simulink model "BlockTypeFrequencyAnalyzerTest"  (Simulink 6.3)
settings: Solver=ode45  StartTime=0.0  StopTime=10.0  RelTol=1e-3
undefined symbols (not defined in the file): DiscIntNeverNeededParam, NumBits1, NumBits2, sigbuilder_block, Slope1, Slope2
libraries: simulink x99
settings Model: LastModifiedBy=deissenb  BufferReuse=off
settings OptimizationCC: BlockReduction=off  InlineParams=on  BufferReuse=off

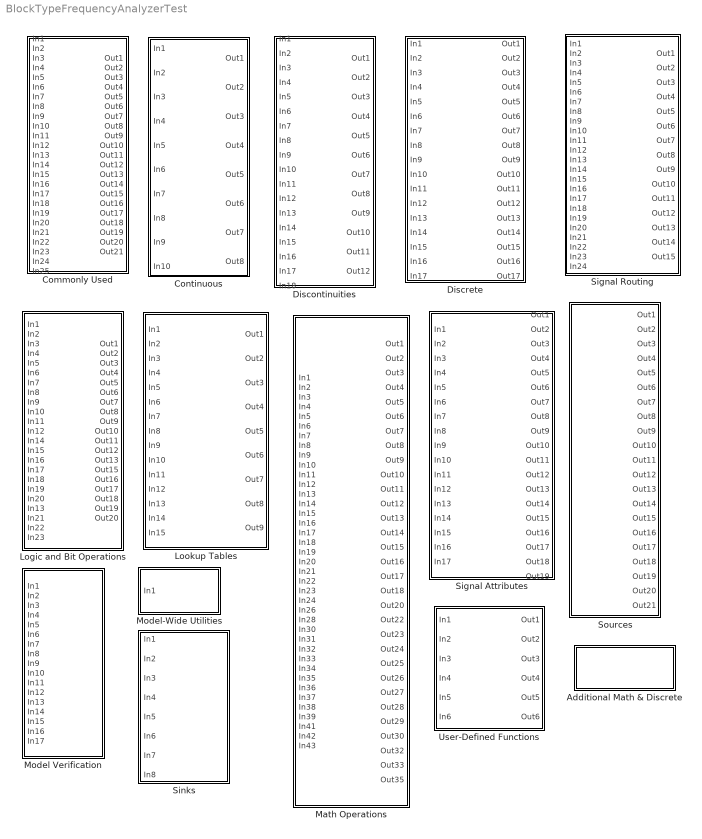
== system BlockTypeFrequencyAnalyzerTest ==
  Additional Math & Discrete : Subsystem
  Commonly Used : Subsystem
  Continuous : Subsystem
  Discontinuities : Subsystem
  Discrete : Subsystem
  Logic and Bit Operations : Subsystem
  Lookup Tables : Subsystem
  Math Operations : Subsystem
  Model Verification : Subsystem
  Model-Wide Utilities : Subsystem
  Signal Attributes : Subsystem
  Signal Routing : Subsystem
  Sinks : Subsystem
  Sources : Subsystem
  User-Defined Functions : Subsystem

== system BlockTypeFrequencyAnalyzerTest/Additional Math & Discrete ==
  Additional Discrete : Subsystem
  Additional Math : Subsystem

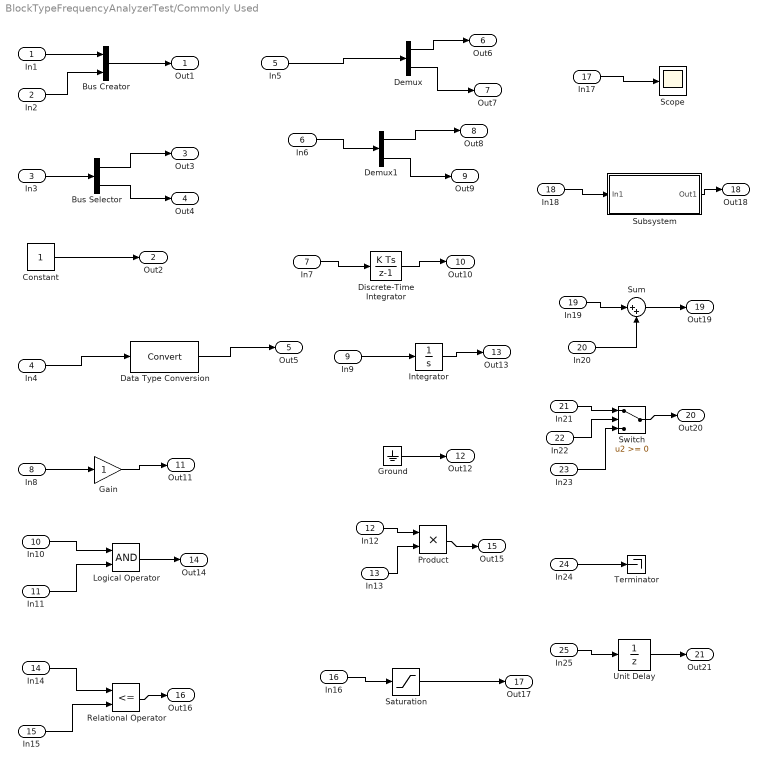
== system BlockTypeFrequencyAnalyzerTest/Commonly Used ==
  In1 : Inport
  In2 : Inport  Port=2
  In3 : Inport  Port=3
  In4 : Inport  Port=4
  In5 : Inport  Port=5
  In6 : Inport  Port=6
  In7 : Inport  Port=7
  In8 : Inport  Port=8
  In9 : Inport  Port=9
  In10 : Inport  Port=10
  In11 : Inport  Port=11
  In12 : Inport  Port=12
  In13 : Inport  Port=13
  In14 : Inport  Port=14
  In15 : Inport  Port=15
  In16 : Inport  Port=16
  In17 : Inport  Port=17
  In18 : Inport  Port=18
  In19 : Inport  Port=19
  In20 : Inport  Port=20
  In21 : Inport  Port=21
  In22 : Inport  Port=22
  In23 : Inport  Port=23
  In24 : Inport  Port=24
  In25 : Inport  Port=25
  Bus Creator : BusCreator  Inputs=2
  Bus Selector : BusSelector  OutputSignals=signal1,signal2
  Constant : Constant
  Data Type Conversion : DataTypeConversion
  Demux : Demux  Outputs=2
  Demux1 : Demux  Outputs=2
  Discrete-Time Integrator : DiscreteIntegrator  ICPrevOutput=DiscIntNeverNeededParam  ICPrevScaledInput=DiscIntNeverNeededParam
  Gain : Gain
  Ground : Ground
  Integrator : Integrator
  Logical Operator : Logic  AllPortsSameDT=off  OutDataTypeMode=Boolean
  Product : Product  RndMeth=Zero
  Relational Operator : RelationalOperator  Operator=<=  LogicOutDataTypeMode=Boolean
  Saturation : Saturate
  Scope : Scope
  Subsystem : Subsystem
  Sum : Sum  Inputs=|++
  Switch : Switch
  Terminator : Terminator
  Unit Delay : UnitDelay
  Out1 : Outport
  Out2 : Outport  Port=2
  Out3 : Outport  Port=3
  Out4 : Outport  Port=4
  Out5 : Outport  Port=5
  Out6 : Outport  Port=6
  Out7 : Outport  Port=7
  Out8 : Outport  Port=8
  Out9 : Outport  Port=9
  Out10 : Outport  Port=10
  Out11 : Outport  Port=11
  Out12 : Outport  Port=12
  Out13 : Outport  Port=13
  Out14 : Outport  Port=14
  Out15 : Outport  Port=15
  Out16 : Outport  Port=16
  Out17 : Outport  Port=17
  Out18 : Outport  Port=18
  Out19 : Outport  Port=19
  Out20 : Outport  Port=20
  Out21 : Outport  Port=21
  wires:
  Unit Delay/1 -> Out21/1
  In25/1 -> Unit Delay/1
  In24/1 -> Terminator/1
  Switch/1 -> Out20/1
  In23/1 -> Switch/3
  In22/1 -> Switch/2
  In21/1 -> Switch/1
  Sum/1 -> Out19/1
  In20/1 -> Sum/2
  In19/1 -> Sum/1
  Subsystem/1(Out1) -> Out18/1
  In18/1 -> Subsystem/1(In1)
  In17/1 -> Scope/1
  Saturation/1 -> Out17/1
  In16/1 -> Saturation/1
  Relational Operator/1 -> Out16/1
  In15/1 -> Relational Operator/2
  In14/1 -> Relational Operator/1
  Product/1 -> Out15/1
  In13/1 -> Product/2
  In12/1 -> Product/1
  Logical Operator/1 -> Out14/1
  In11/1 -> Logical Operator/2
  In10/1 -> Logical Operator/1
  Integrator/1 -> Out13/1
  In9/1 -> Integrator/1
  Ground/1 -> Out12/1
  Gain/1 -> Out11/1
  In8/1 -> Gain/1
  Discrete-Time Integrator/1 -> Out10/1
  In7/1 -> Discrete-Time Integrator/1
  Demux1/2 -> Out9/1
  Demux1/1 -> Out8/1
  In6/1 -> Demux1/1
  Demux/2 -> Out7/1
  Demux/1 -> Out6/1
  In5/1 -> Demux/1
  Data Type Conversion/1 -> Out5/1
  In4/1 -> Data Type Conversion/1
  Bus Selector/2 -> Out4/1
  Bus Selector/1 -> Out3/1
  In3/1 -> Bus Selector/1
  Constant/1 -> Out2/1
  Bus Creator/1 -> Out1/1
  In2/1 -> Bus Creator/2
  In1/1 -> Bus Creator/1

== system BlockTypeFrequencyAnalyzerTest/Continuous ==
  In1 : Inport
  In2 : Inport  Port=2
  In3 : Inport  Port=3
  In4 : Inport  Port=4
  In5 : Inport  Port=5
  In6 : Inport  Port=6
  In7 : Inport  Port=7
  In8 : Inport  Port=8
  In9 : Inport  Port=9
  In10 : Inport  Port=10
  Derivative : Derivative
  Integrator : Integrator
  State-Space : StateSpace
  Transfer Fcn : TransferFcn  Denominator=[1 1]
  Transport Delay : TransportDelay
  Variable Time Delay : VariableTransportDelay  MaximumDelay=10
  Variable Transport Delay : VariableTransportDelay  VariableDelayType=Variable transport delay  MaximumDelay=10
  Zero-Pole : ZeroPole  Poles=[0 -1]
  Out1 : Outport
  Out2 : Outport  Port=2
  Out3 : Outport  Port=3
  Out4 : Outport  Port=4
  Out5 : Outport  Port=5
  Out6 : Outport  Port=6
  Out7 : Outport  Port=7
  Out8 : Outport  Port=8
  wires:
  In1/1 -> Derivative/1
  In2/1 -> Integrator/1
  In3/1 -> State-Space/1
  In4/1 -> Transfer Fcn/1
  In5/1 -> Transport Delay/1
  In6/1 -> Variable Time Delay/1
  In7/1 -> Variable Time Delay/2
  In8/1 -> Variable Transport Delay/1
  In9/1 -> Variable Transport Delay/2
  In10/1 -> Zero-Pole/1
  Derivative/1 -> Out1/1
  Integrator/1 -> Out2/1
  State-Space/1 -> Out3/1
  Transfer Fcn/1 -> Out4/1
  Transport Delay/1 -> Out5/1
  Variable Time Delay/1 -> Out6/1
  Variable Transport Delay/1 -> Out7/1
  Zero-Pole/1 -> Out8/1

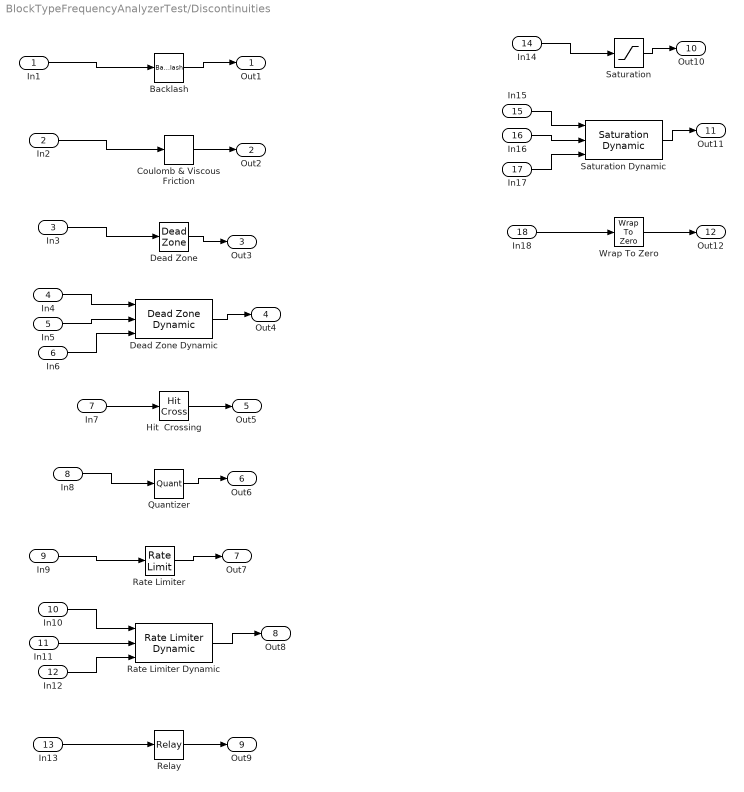
== system BlockTypeFrequencyAnalyzerTest/Discontinuities ==
  In1 : Inport
  In2 : Inport  Port=2
  In3 : Inport  Port=3
  In4 : Inport  Port=4
  In5 : Inport  Port=5
  In6 : Inport  Port=6
  In7 : Inport  Port=7
  In8 : Inport  Port=8
  In9 : Inport  Port=9
  In10 : Inport  Port=10
  In11 : Inport  Port=11
  In12 : Inport  Port=12
  In13 : Inport  Port=13
  In14 : Inport  Port=14
  In15 : Inport  Port=15
  In16 : Inport  Port=16
  In17 : Inport  Port=17
  In18 : Inport  Port=18
  Backlash : Backlash
  Coulomb & Viscous Friction : simulink/Discontinuities/Coulomb & Viscous Friction  offset=[1 3 2 0]  gain=1
  Dead Zone : DeadZone  SaturateOnIntegerOverflow=on
  Dead Zone Dynamic : simulink/Discontinuities/Dead Zone Dynamic
  Hit  Crossing : HitCross
  Quantizer : Quantizer
  Rate Limiter : RateLimiter  SampleTimeMode=inherited
  Rate Limiter Dynamic : simulink/Discontinuities/Rate Limiter Dynamic
  Relay : Relay
  Saturation : Saturate
  Saturation Dynamic : simulink/Discontinuities/Saturation Dynamic
  Wrap To Zero : simulink/Discontinuities/Wrap To Zero  Threshold=255
  Out1 : Outport
  Out2 : Outport  Port=2
  Out3 : Outport  Port=3
  Out4 : Outport  Port=4
  Out5 : Outport  Port=5
  Out6 : Outport  Port=6
  Out7 : Outport  Port=7
  Out8 : Outport  Port=8
  Out9 : Outport  Port=9
  Out10 : Outport  Port=10
  Out11 : Outport  Port=11
  Out12 : Outport  Port=12
  wires:
  In1/1 -> Backlash/1
  In2/1 -> Coulomb & Viscous Friction/1
  In3/1 -> Dead Zone/1
  In4/1 -> Dead Zone Dynamic/1
  In5/1 -> Dead Zone Dynamic/2
  In6/1 -> Dead Zone Dynamic/3
  In7/1 -> Hit  Crossing/1
  In8/1 -> Quantizer/1
  In9/1 -> Rate Limiter/1
  In10/1 -> Rate Limiter Dynamic/1
  In11/1 -> Rate Limiter Dynamic/2
  In12/1 -> Rate Limiter Dynamic/3
  In13/1 -> Relay/1
  In14/1 -> Saturation/1
  In15/1 -> Saturation Dynamic/1
  In16/1 -> Saturation Dynamic/2
  In17/1 -> Saturation Dynamic/3
  In18/1 -> Wrap To Zero/1
  Backlash/1 -> Out1/1
  Coulomb & Viscous Friction/1 -> Out2/1
  Dead Zone/1 -> Out3/1
  Dead Zone Dynamic/1 -> Out4/1
  Hit  Crossing/1 -> Out5/1
  Quantizer/1 -> Out6/1
  Rate Limiter/1 -> Out7/1
  Rate Limiter Dynamic/1 -> Out8/1
  Relay/1 -> Out9/1
  Saturation/1 -> Out10/1
  Saturation Dynamic/1 -> Out11/1
  Wrap To Zero/1 -> Out12/1

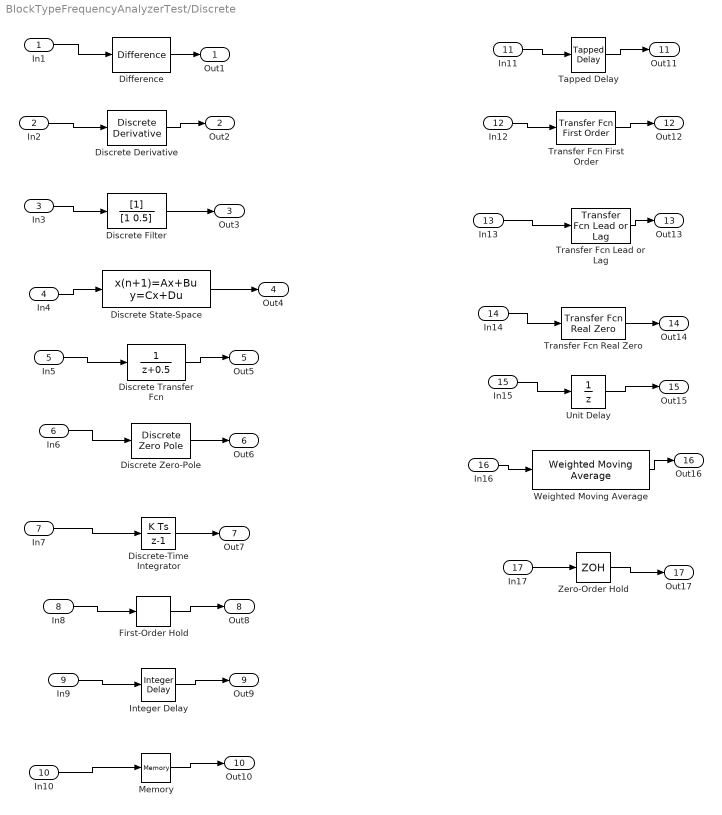
== system BlockTypeFrequencyAnalyzerTest/Discrete ==
  In1 : Inport
  In2 : Inport  Port=2
  In3 : Inport  Port=3
  In4 : Inport  Port=4
  In5 : Inport  Port=5
  In6 : Inport  Port=6
  In7 : Inport  Port=7
  In8 : Inport  Port=8
  In9 : Inport  Port=9
  In10 : Inport  Port=10
  In11 : Inport  Port=11
  In12 : Inport  Port=12
  In13 : Inport  Port=13
  In14 : Inport  Port=14
  In15 : Inport  Port=15
  In16 : Inport  Port=16
  In17 : Inport  Port=17
  Difference : simulink/Discrete/Difference  ICPrevInput=0.0  OutDataType=sfix(16)  OutScaling=2^-10  DoSatur=off
  Discrete Transfer Fcn : DiscreteTransferFcn
  Discrete Zero-Pole : DiscreteZeroPole  Poles=[0 0.5]  Gain=1
  Discrete Derivative : simulink/Discrete/Discrete Derivative  gainval=1.0  ICPrevScaledInput=0.0  OutDataType=sfix(16)  OutScaling=2^-10  DoSatur=off
  Discrete Filter : DiscreteFilter  Denominator=[1 0.5]
  Discrete State-Space : DiscreteStateSpace
  Discrete-Time Integrator : DiscreteIntegrator  ICPrevOutput=DiscIntNeverNeededParam  ICPrevScaledInput=DiscIntNeverNeededParam
  First-Order Hold : simulink/Discrete/First-Order Hold  DisableCoverage=on  Ts=1
  Integer Delay : simulink/Discrete/Integer Delay  vinit=0.0  samptime=-1  NumDelays=4
  Memory : Memory
  Tapped Delay : simulink/Discrete/Tapped Delay  vinit=0.0  samptime=-1  NumDelays=4  DelayOrder=Oldest  includeCurrent=off
  Transfer Fcn First Order : simulink/Discrete/Transfer Fcn First Order  PoleZ=0.95  ICPrevOutput=0.0  DoSatur=off
  Transfer Fcn Lead or Lag : simulink/Discrete/Transfer Fcn Lead or Lag  PoleZ=0.95  ZeroZ=0.75  ICPrevOutput=0.0  ICPrevInput=0.0  DoSatur=off
  Transfer Fcn Real Zero : simulink/Discrete/Transfer Fcn Real Zero  ZeroZ=0.75  ICPrevInput=0.0  DoSatur=off
  Unit Delay : UnitDelay
  Weighted Moving Average : simulink/Discrete/Weighted Moving Average  mgainval=[0.1:0.1:1 0.9:-0.1:0.1]  vinit=0.0  samptime=-1  GainDataType=sfix( 16 )  MatRadixGroup=Best Precision: Matrix-wise  GainScaling=2^-10  OutDataType=sfix(16)  OutScaling=2^-10  DoSatur=off
  Zero-Order Hold : ZeroOrderHold
  Out1 : Outport
  Out2 : Outport  Port=2
  Out3 : Outport  Port=3
  Out4 : Outport  Port=4
  Out5 : Outport  Port=5
  Out6 : Outport  Port=6
  Out7 : Outport  Port=7
  Out8 : Outport  Port=8
  Out9 : Outport  Port=9
  Out10 : Outport  Port=10
  Out11 : Outport  Port=11
  Out12 : Outport  Port=12
  Out13 : Outport  Port=13
  Out14 : Outport  Port=14
  Out15 : Outport  Port=15
  Out16 : Outport  Port=16
  Out17 : Outport  Port=17
  wires:
  In1/1 -> Difference/1
  In2/1 -> Discrete Derivative/1
  In3/1 -> Discrete Filter/1
  In4/1 -> Discrete State-Space/1
  In5/1 -> Discrete Transfer Fcn/1
  In6/1 -> Discrete Zero-Pole/1
  In7/1 -> Discrete-Time Integrator/1
  In8/1 -> First-Order Hold/1
  In9/1 -> Integer Delay/1
  In10/1 -> Memory/1
  In11/1 -> Tapped Delay/1
  In12/1 -> Transfer Fcn First Order/1
  In13/1 -> Transfer Fcn Lead or Lag/1
  In14/1 -> Transfer Fcn Real Zero/1
  In15/1 -> Unit Delay/1
  In16/1 -> Weighted Moving Average/1
  In17/1 -> Zero-Order Hold/1
  Difference/1 -> Out1/1
  Discrete Derivative/1 -> Out2/1
  Discrete Filter/1 -> Out3/1
  Discrete State-Space/1 -> Out4/1
  Discrete Transfer Fcn/1 -> Out5/1
  Discrete Zero-Pole/1 -> Out6/1
  Discrete-Time Integrator/1 -> Out7/1
  First-Order Hold/1 -> Out8/1
  Integer Delay/1 -> Out9/1
  Memory/1 -> Out10/1
  Tapped Delay/1 -> Out11/1
  Transfer Fcn First Order/1 -> Out12/1
  Transfer Fcn Lead or Lag/1 -> Out13/1
  Transfer Fcn Real Zero/1 -> Out14/1
  Unit Delay/1 -> Out15/1
  Weighted Moving Average/1 -> Out16/1
  Zero-Order Hold/1 -> Out17/1

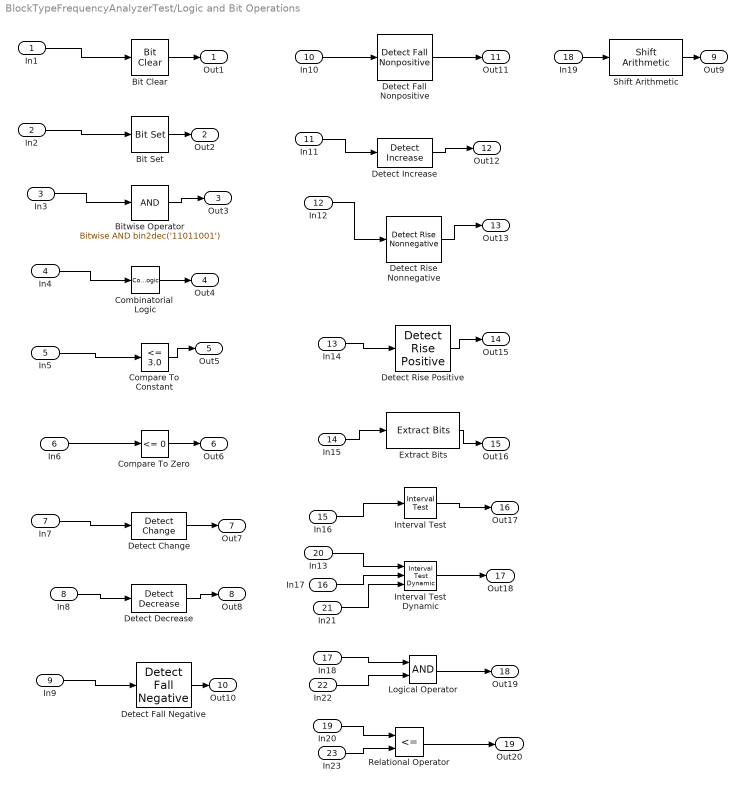
== system BlockTypeFrequencyAnalyzerTest/Logic and Bit Operations ==
  In1 : Inport
  In2 : Inport  Port=2
  In3 : Inport  Port=3
  In4 : Inport  Port=4
  In5 : Inport  Port=5
  In6 : Inport  Port=6
  In7 : Inport  Port=7
  In8 : Inport  Port=8
  In9 : Inport  Port=9
  In10 : Inport  Port=10
  In11 : Inport  Port=11
  In12 : Inport  Port=12
  In14 : Inport  Port=13
  In15 : Inport  Port=14
  In16 : Inport  Port=15
  In17 : Inport  Port=16
  In18 : Inport  Port=17
  In19 : Inport  Port=18
  In20 : Inport  Port=19
  In13 : Inport  Port=20
  In21 : Inport  Port=21
  In22 : Inport  Port=22
  In23 : Inport  Port=23
  Bit Clear : simulink/Logic and Bit Operations/Bit Clear  iBit=0
  Bit Set : simulink/Logic and Bit Operations/Bit Set  iBit=0
  Bitwise Operator : simulink/Logic and Bit Operations/Bitwise Operator  logicop=AND  UseBitMask=on  BitMask=bin2dec('11011001')  BitMaskRealWorld=Stored Integer
  Combinatorial  Logic : CombinatorialLogic
  Compare To Constant : simulink/Logic and Bit Operations/Compare To Constant  relop=<=  const=3.0  LogicOutDataTypeMode=uint8  ZeroCross=off
  Compare To Zero : simulink/Logic and Bit Operations/Compare To Zero  relop=<=  LogicOutDataTypeMode=uint8  ZeroCross=off
  Detect Change : simulink/Logic and Bit Operations/Detect Change  vinit=0
  Detect Decrease : simulink/Logic and Bit Operations/Detect Decrease  vinit=0.0
  Detect Increase : simulink/Logic and Bit Operations/Detect Increase  vinit=0.0
  Detect Fall Negative : simulink/Logic and Bit Operations/Detect Fall Negative  vinit=0
  Detect Fall Nonpositive : simulink/Logic and Bit Operations/Detect Fall Nonpositive  vinit=0
  Detect Rise Nonnegative : simulink/Logic and Bit Operations/Detect Rise Nonnegative  vinit=0
  Detect Rise Positive : simulink/Logic and Bit Operations/Detect Rise Positive  vinit=0
  Extract Bits : simulink/Logic and Bit Operations/Extract Bits  bitsToExtract=Upper half  numBits=8  bitIdxRange=[0 7]  outScalingMode=Preserve fixed-point scaling
  Interval Test : simulink/Logic and Bit Operations/Interval Test  IntervalClosedRight=on  uplimit=0.5  IntervalClosedLeft=on  lowlimit=-0.5  LogicOutDataTypeMode=boolean
  Interval Test Dynamic : simulink/Logic and Bit Operations/Interval Test Dynamic  IntervalClosedRight=on  IntervalClosedLeft=on  LogicOutDataTypeMode=boolean
  Logical Operator : Logic  AllPortsSameDT=off  OutDataTypeMode=Boolean
  Relational Operator : RelationalOperator  Operator=<=  LogicOutDataTypeMode=Boolean
  Shift Arithmetic : simulink/Logic and Bit Operations/Shift Arithmetic  nBitShiftRight=8  nBinPtShiftRight=0
  Out1 : Outport
  Out2 : Outport  Port=2
  Out3 : Outport  Port=3
  Out4 : Outport  Port=4
  Out5 : Outport  Port=5
  Out6 : Outport  Port=6
  Out7 : Outport  Port=7
  Out8 : Outport  Port=8
  Out9 : Outport  Port=9
  Out10 : Outport  Port=10
  Out11 : Outport  Port=11
  Out12 : Outport  Port=12
  Out13 : Outport  Port=13
  Out15 : Outport  Port=14
  Out16 : Outport  Port=15
  Out17 : Outport  Port=16
  Out18 : Outport  Port=17
  Out19 : Outport  Port=18
  Out20 : Outport  Port=19
  wires:
  In1/1 -> Bit Clear/1
  In2/1 -> Bit Set/1
  In3/1 -> Bitwise Operator/1
  In4/1 -> Combinatorial  Logic/1
  In5/1 -> Compare To Constant/1
  In6/1 -> Compare To Zero/1
  In7/1 -> Detect Change/1
  In8/1 -> Detect Decrease/1
  In9/1 -> Detect Fall Negative/1
  Bit Clear/1 -> Out1/1
  Bit Set/1 -> Out2/1
  Bitwise Operator/1 -> Out3/1
  Combinatorial  Logic/1 -> Out4/1
  Compare To Constant/1 -> Out5/1
  Compare To Zero/1 -> Out6/1
  Detect Change/1 -> Out7/1
  Detect Decrease/1 -> Out8/1
  Detect Fall Negative/1 -> Out10/1
  In10/1 -> Detect Fall Nonpositive/1
  In11/1 -> Detect Increase/1
  In12/1 -> Detect Rise Nonnegative/1
  In14/1 -> Detect Rise Positive/1
  In15/1 -> Extract Bits/1
  In16/1 -> Interval Test/1
  In17/1 -> Interval Test Dynamic/2
  In13/1 -> Interval Test Dynamic/1
  In21/1 -> Interval Test Dynamic/3
  In18/1 -> Logical Operator/1
  In22/1 -> Logical Operator/2
  In20/1 -> Relational Operator/1
  In23/1 -> Relational Operator/2
  Detect Fall Nonpositive/1 -> Out11/1
  Detect Increase/1 -> Out12/1
  Detect Rise Nonnegative/1 -> Out13/1
  Detect Rise Positive/1 -> Out15/1
  Extract Bits/1 -> Out16/1
  Interval Test/1 -> Out17/1
  Interval Test Dynamic/1 -> Out18/1
  Logical Operator/1 -> Out19/1
  Relational Operator/1 -> Out20/1
  In19/1 -> Shift Arithmetic/1
  Shift Arithmetic/1 -> Out9/1

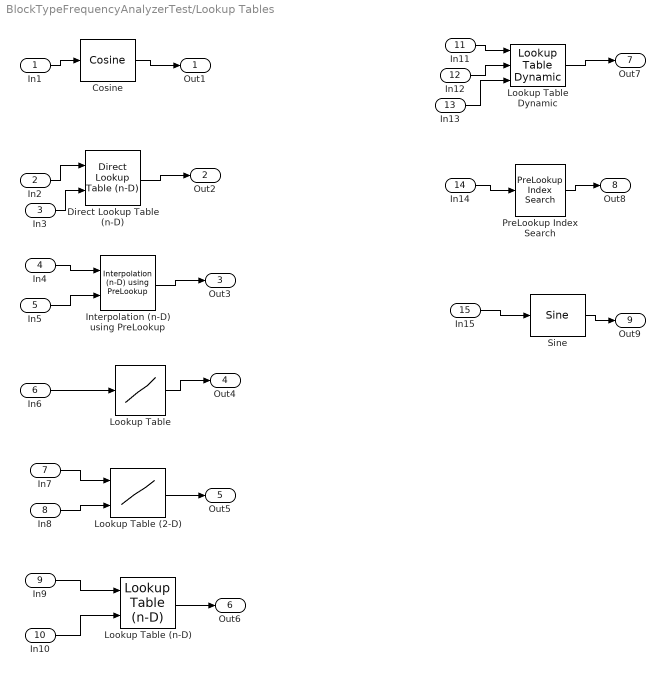
== system BlockTypeFrequencyAnalyzerTest/Lookup Tables ==
  In1 : Inport
  In2 : Inport  Port=2
  In3 : Inport  Port=3
  In4 : Inport  Port=4
  In5 : Inport  Port=5
  In6 : Inport  Port=6
  In7 : Inport  Port=7
  In8 : Inport  Port=8
  In9 : Inport  Port=9
  In10 : Inport  Port=10
  In11 : Inport  Port=11
  In12 : Inport  Port=12
  In13 : Inport  Port=13
  In14 : Inport  Port=14
  In15 : Inport  Port=15
  Cosine : simulink/Lookup Tables/Cosine  Formula=cos(2*pi*u)  NumDataPoints=(2^5)+1  OutputWordLength=16
  Direct Lookup Table (n-D) : simulink/Lookup Tables/Direct Lookup Table (n-D)  maskTabDims=2  explicitNumDims=1  outDims=Element  tabIsInput=off  mxTable=[4 5 6;16 19 20;10 18 23]  clipFlag=Warning
  Interpolation (n-D) using PreLookup : simulink/Lookup Tables/Interpolation (n-D) using PreLookup  numDimsPopupSelect=2  explicitNumDims=2  table=sqrt([1:10]'*[1:10])  interpMethod=Linear  extrapMethod=Linear  rangeErrorMode=None  NumSelectionDims=0
  Lookup Table Dynamic : simulink/Lookup Tables/Lookup Table Dynamic  LookUpMeth=Interpolation-Use End Values  OutputDataTypeScalingMode=Specify via dialog  OutDataType=float('double')  OutScaling=2^-10  DoSatur=off
  Lookup Table (2-D) : Lookup2D  RowIndex=[1:3]  ColumnIndex=[1:3]  OutputValues=[4 5 6;16 19 20;10 18 23]
  Lookup Table (n-D) : simulink/Lookup Tables/Lookup Table (n-D)  numDimsPopupSelect=2  bp1=[10,22,31]  bp2=[10,22,31]  bp3=[1:3]  bp4=[1:3]  bpcell={ [1:3], [1:3] }  explicitNumDims=2  searchMode=Binary Search  cacheBpFlag=off  vectorInputFlag=off  tableData=[4 5 6;16 19 20;10 18 23]  interpMethod=Linear  extrapMethod=Linear  rangeErrorMode=None
  Lookup Table : Lookup  InputValues=[-5:5]  OutputValues=tanh([-5:5])
  PreLookup Index Search : simulink/Lookup Tables/PreLookup Index Search  bpData=[10:10:100]  searchMode=Binary Search  cacheBpFlag=off  outputFlag=off  IndexDataType=uint32  extrapMode=Linear Extrapolation  rangeErrorMode=None
  Sine : simulink/Lookup Tables/Sine  Formula=sin(2*pi*u)  NumDataPoints=(2^5)+1  OutputWordLength=16
  Out1 : Outport
  Out2 : Outport  Port=2
  Out3 : Outport  Port=3
  Out4 : Outport  Port=4
  Out5 : Outport  Port=5
  Out6 : Outport  Port=6
  Out7 : Outport  Port=7
  Out8 : Outport  Port=8
  Out9 : Outport  Port=9
  wires:
  In1/1 -> Cosine/1
  In2/1 -> Direct Lookup Table (n-D)/1
  In3/1 -> Direct Lookup Table (n-D)/2
  In4/1 -> Interpolation (n-D) using PreLookup/1
  In5/1 -> Interpolation (n-D) using PreLookup/2
  In6/1 -> Lookup Table/1
  In7/1 -> Lookup Table (2-D)/1
  In8/1 -> Lookup Table (2-D)/2
  In9/1 -> Lookup Table (n-D)/1
  In10/1 -> Lookup Table (n-D)/2
  In11/1 -> Lookup Table Dynamic/1
  In12/1 -> Lookup Table Dynamic/2
  In13/1 -> Lookup Table Dynamic/3
  In14/1 -> PreLookup Index Search/1
  In15/1 -> Sine/1
  Cosine/1 -> Out1/1
  Direct Lookup Table (n-D)/1 -> Out2/1
  Interpolation (n-D) using PreLookup/1 -> Out3/1
  Lookup Table/1 -> Out4/1
  Lookup Table (2-D)/1 -> Out5/1
  Lookup Table (n-D)/1 -> Out6/1
  Lookup Table Dynamic/1 -> Out7/1
  PreLookup Index Search/1 -> Out8/1
  Sine/1 -> Out9/1

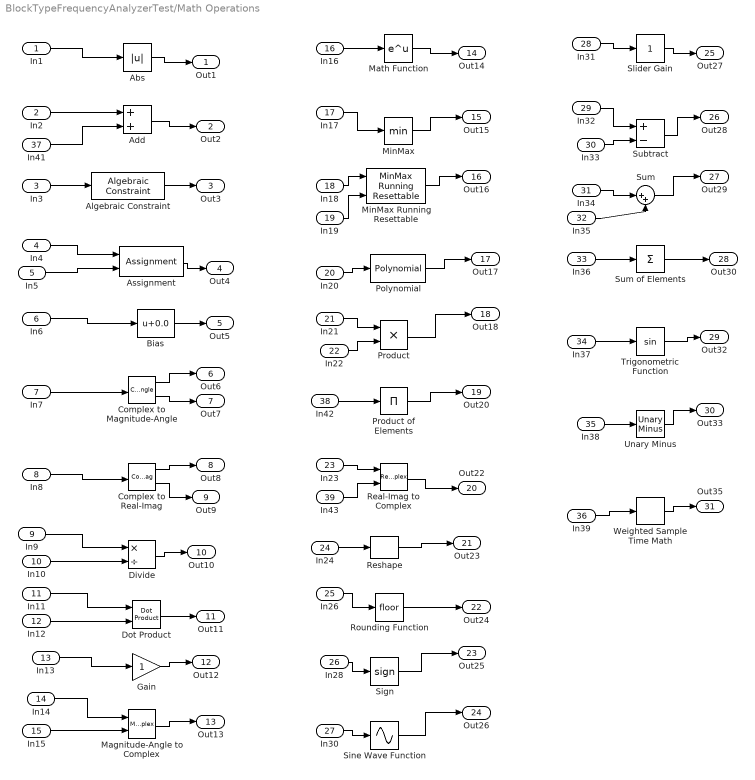
== system BlockTypeFrequencyAnalyzerTest/Math Operations ==
  In1 : Inport
  In2 : Inport  Port=2
  In3 : Inport  Port=3
  In4 : Inport  Port=4
  In5 : Inport  Port=5
  In6 : Inport  Port=6
  In7 : Inport  Port=7
  In8 : Inport  Port=8
  In9 : Inport  Port=9
  In10 : Inport  Port=10
  In11 : Inport  Port=11
  In12 : Inport  Port=12
  In13 : Inport  Port=13
  In14 : Inport  Port=14
  In15 : Inport  Port=15
  In16 : Inport  Port=16
  In17 : Inport  Port=17
  In18 : Inport  Port=18
  In19 : Inport  Port=19
  In20 : Inport  Port=20
  In21 : Inport  Port=21
  In22 : Inport  Port=22
  In23 : Inport  Port=23
  In24 : Inport  Port=24
  In26 : Inport  Port=25
  In28 : Inport  Port=26
  In30 : Inport  Port=27
  In31 : Inport  Port=28
  In32 : Inport  Port=29
  In33 : Inport  Port=30
  In34 : Inport  Port=31
  In35 : Inport  Port=32
  In36 : Inport  Port=33
  In37 : Inport  Port=34
  In38 : Inport  Port=35
  In39 : Inport  Port=36
  In41 : Inport  Port=37
  In42 : Inport  Port=38
  In43 : Inport  Port=39
  Abs : Abs
  Add : Sum  OutScaling=2^-10
  Algebraic Constraint : simulink/Math Operations/Algebraic Constraint  z0=0
  Assignment : Assignment
  Bias : Bias  Bias=0.0
  Complex to Magnitude-Angle : ComplexToMagnitudeAngle
  Complex to Real-Imag : ComplexToRealImag
  Divide : Product  Inputs=*/  OutScaling=2^-10
  Dot Product : simulink/Math Operations/Dot Product  InputSameDT=on  OutDataType=sfix(16)  OutScaling=2^-10  DoSatur=off
  Gain : Gain
  Magnitude-Angle to Complex : MagnitudeAngleToComplex
  Math Function : Math  SaturateOnIntegerOverflow=on
  MinMax : MinMax
  MinMax Running Resettable : simulink/Math Operations/MinMax Running Resettable  Function=min  vinit=0.0
  Polynomial : simulink/Math Operations/Polynomial  coefs=[ +2.081618890e-019, -1.441693666e-014, +4.719686976e-010, -8.536869453e-006, +1.621573104e-001, -8.087801117e+001 ]
  Product : Product  RndMeth=Zero
  Product of Elements : Product  Inputs=*  OutScaling=2^-10
  Real-Imag to Complex : RealImagToComplex
  Reshape : simulink/Math Operations/Reshape  OutputDimensionality=1-D array  OutputDimensions=[1,1]
  Rounding Function : Rounding
  Sign : Signum
  Sine Wave Function : Sin  TimeSource=Use external signal  SampleTime=0
  Slider Gain : simulink/Math Operations/Slider Gain  low=0  gain=1  high=2
  Subtract : Sum  Inputs=+-  OutScaling=2^-10
  Sum : Sum  Inputs=|++
  Sum of Elements : Sum  Inputs=+  OutScaling=2^-10
  Trigonometric Function : Trigonometry
  Unary Minus : simulink/Math Operations/Unary Minus  DoSatur=off
  Weighted Sample Time Math : simulink/Math Operations/Weighted Sample Time Math  TsampMathOp=+  weightValue=1.0  TsampMathImp=Online Calculations  DoSatur=off
  Out1 : Outport
  Out2 : Outport  Port=2
  Out3 : Outport  Port=3
  Out4 : Outport  Port=4
  Out5 : Outport  Port=5
  Out6 : Outport  Port=6
  Out7 : Outport  Port=7
  Out8 : Outport  Port=8
  Out9 : Outport  Port=9
  Out10 : Outport  Port=10
  Out11 : Outport  Port=11
  Out12 : Outport  Port=12
  Out13 : Outport  Port=13
  Out14 : Outport  Port=14
  Out15 : Outport  Port=15
  Out16 : Outport  Port=16
  Out17 : Outport  Port=17
  Out18 : Outport  Port=18
  Out20 : Outport  Port=19
  Out22 : Outport  Port=20
  Out23 : Outport  Port=21
  Out24 : Outport  Port=22
  Out25 : Outport  Port=23
  Out26 : Outport  Port=24
  Out27 : Outport  Port=25
  Out28 : Outport  Port=26
  Out29 : Outport  Port=27
  Out30 : Outport  Port=28
  Out32 : Outport  Port=29
  Out33 : Outport  Port=30
  Out35 : Outport  Port=31
  wires:
  In1/1 -> Abs/1
  In2/1 -> Add/1
  In41/1 -> Add/2
  In3/1 -> Algebraic Constraint/1
  In4/1 -> Assignment/1
  In5/1 -> Assignment/2
  In6/1 -> Bias/1
  In7/1 -> Complex to Magnitude-Angle/1
  In8/1 -> Complex to Real-Imag/1
  In9/1 -> Divide/1
  In10/1 -> Divide/2
  In11/1 -> Dot Product/1
  In12/1 -> Dot Product/2
  In13/1 -> Gain/1
  In14/1 -> Magnitude-Angle to Complex/1
  In15/1 -> Magnitude-Angle to Complex/2
  Abs/1 -> Out1/1
  Add/1 -> Out2/1
  Algebraic Constraint/1 -> Out3/1
  Assignment/1 -> Out4/1
  Bias/1 -> Out5/1
  Complex to Magnitude-Angle/1 -> Out6/1
  Complex to Magnitude-Angle/2 -> Out7/1
  Complex to Real-Imag/1 -> Out8/1
  Complex to Real-Imag/2 -> Out9/1
  Divide/1 -> Out10/1
  Dot Product/1 -> Out11/1
  Gain/1 -> Out12/1
  Magnitude-Angle to Complex/1 -> Out13/1
  In16/1 -> Math Function/1
  Math Function/1 -> Out14/1
  In17/1 -> MinMax/1
  MinMax/1 -> Out15/1
  In18/1 -> MinMax Running Resettable/1
  In19/1 -> MinMax Running Resettable/2
  MinMax Running Resettable/1 -> Out16/1
  In20/1 -> Polynomial/1
  Polynomial/1 -> Out17/1
  In21/1 -> Product/1
  In22/1 -> Product/2
  Product/1 -> Out18/1
  In42/1 -> Product of Elements/1
  Product of Elements/1 -> Out20/1
  In23/1 -> Real-Imag to Complex/1
  In43/1 -> Real-Imag to Complex/2
  Real-Imag to Complex/1 -> Out22/1
  In24/1 -> Reshape/1
  Reshape/1 -> Out23/1
  In26/1 -> Rounding Function/1
  Rounding Function/1 -> Out24/1
  In28/1 -> Sign/1
  Sign/1 -> Out25/1
  In30/1 -> Sine Wave Function/1
  Sine Wave Function/1 -> Out26/1
  In31/1 -> Slider Gain/1
  Slider Gain/1 -> Out27/1
  In32/1 -> Subtract/1
  Subtract/1 -> Out28/1
  In33/1 -> Subtract/2
  In34/1 -> Sum/1
  In35/1 -> Sum/2
  Sum/1 -> Out29/1
  In36/1 -> Sum of Elements/1
  Sum of Elements/1 -> Out30/1
  In37/1 -> Trigonometric Function/1
  Trigonometric Function/1 -> Out32/1
  In38/1 -> Unary Minus/1
  Unary Minus/1 -> Out33/1
  In39/1 -> Weighted Sample Time Math/1
  Weighted Sample Time Math/1 -> Out35/1

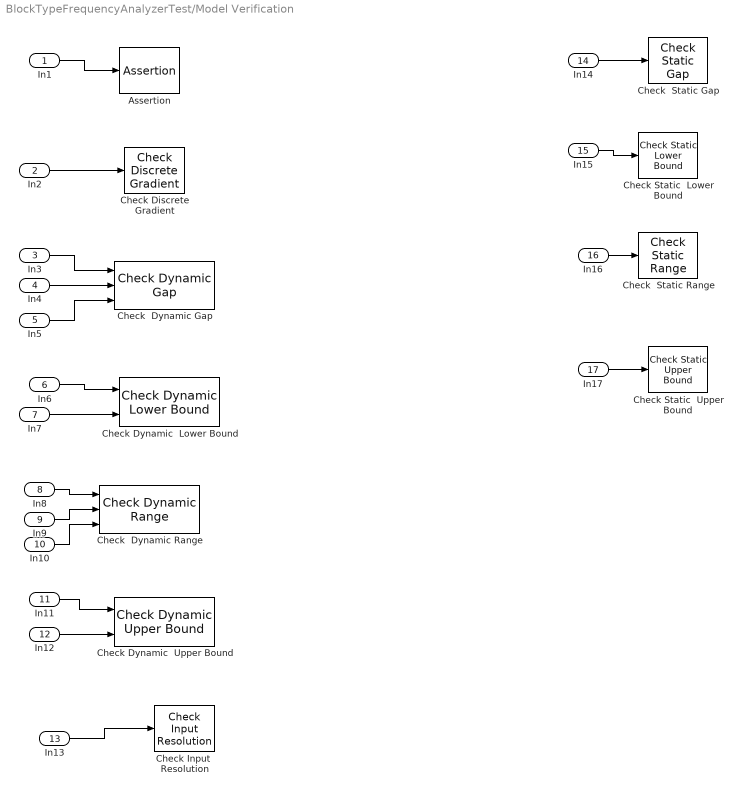
== system BlockTypeFrequencyAnalyzerTest/Model Verification ==
  In1 : Inport
  In2 : Inport  Port=2
  In3 : Inport  Port=3
  In4 : Inport  Port=4
  In5 : Inport  Port=5
  In6 : Inport  Port=6
  In7 : Inport  Port=7
  In8 : Inport  Port=8
  In9 : Inport  Port=9
  In10 : Inport  Port=10
  In11 : Inport  Port=11
  In12 : Inport  Port=12
  In13 : Inport  Port=13
  In14 : Inport  Port=14
  In15 : Inport  Port=15
  In16 : Inport  Port=16
  In17 : Inport  Port=17
  Assertion : Assertion
  Check Discrete Gradient : simulink/Model Verification/Check Discrete Gradient  Description=| du / dt | < 1  gradient=1  enabled=on  stopWhenAssertionFail=on  export=off  icon=graphic
  Check  Dynamic Gap : simulink/Model Verification/Check  Dynamic Gap  Description=sig < min || max < sig  enabled=on  stopWhenAssertionFail=on  export=off  icon=graphic
  Check  Dynamic Range : simulink/Model Verification/Check  Dynamic Range  Description=min < sig < max  enabled=on  stopWhenAssertionFail=on  export=off  icon=graphic
  Check  Static Gap : simulink/Model Verification/Check  Static Gap  Description=u <= 0 || 100 <= u  max=100  max_included=on  min=0  min_included=on  enabled=on  stopWhenAssertionFail=on  export=off  icon=graphic
  Check  Static Range : simulink/Model Verification/Check  Static Range  Description=0 <= u <= 100  max=100  max_included=on  min=0  min_included=on  enabled=on  stopWhenAssertionFail=on  export=off  icon=graphic
  Check Dynamic  Lower Bound : simulink/Model Verification/Check Dynamic  Lower Bound  Description=min < sig  Enabled=on  stopWhenAssertionFail=on  export=off  icon=graphic
  Check Dynamic  Upper Bound : simulink/Model Verification/Check Dynamic  Upper Bound  Description=sig < max  enabled=on  stopWhenAssertionFail=on  export=off  icon=graphic
  Check Input  Resolution : simulink/Model Verification/Check Input  Resolution  Description=-Inf < u < +Inf  resolution=1  enabled=on  stopWhenAssertionFail=on  export=off
  Check Static  Lower Bound : simulink/Model Verification/Check Static  Lower Bound  Description=0 <= u  min=0  min_included=on  enabled=on  stopWhenAssertionFail=on  export=off  icon=graphic
  Check Static  Upper Bound : simulink/Model Verification/Check Static  Upper Bound  Description=u <= 0  max=0  max_included=on  enabled=on  stopWhenAssertionFail=on  export=off  icon=graphic
  wires:
  In1/1 -> Assertion/1
  In2/1 -> Check Discrete Gradient/1
  In3/1 -> Check  Dynamic Gap/1
  In4/1 -> Check  Dynamic Gap/2
  In5/1 -> Check  Dynamic Gap/3
  In6/1 -> Check Dynamic  Lower Bound/1
  In7/1 -> Check Dynamic  Lower Bound/2
  In8/1 -> Check  Dynamic Range/1
  In9/1 -> Check  Dynamic Range/2
  In10/1 -> Check  Dynamic Range/3
  In11/1 -> Check Dynamic  Upper Bound/1
  In12/1 -> Check Dynamic  Upper Bound/2
  In13/1 -> Check Input  Resolution/1
  In14/1 -> Check  Static Gap/1
  In15/1 -> Check Static  Lower Bound/1
  In16/1 -> Check  Static Range/1
  In17/1 -> Check Static  Upper Bound/1

== system BlockTypeFrequencyAnalyzerTest/Model-Wide Utilities ==
  In1 : Inport
  Block Support Table : simulink/Model-Wide Utilities/Block Support Table
  DocBlock : simulink/Model-Wide Utilities/DocBlock  DocumentType=Text
  Model Info : simulink/Model-Wide Utilities/Model Info  InitialBlockCM=None  BlockCM=None  Frame=on  DisplayStringWithTags=Model Info  HorizontalTextAlignment=Center  LeftAlignmentValue=0.5  SourceBlockDiagram=ports  TagMaxNumber=20
  Timed-Based Linearization : simulink/Model-Wide Utilities/Timed-Based Linearization  LinearizationTime=1  SampleTime=0
  Trigger-Based Linearization : simulink/Model-Wide Utilities/Trigger-Based Linearization  TriggerType=rising  SampleTime=0
  wires:
  In1/1 -> Trigger-Based Linearization/Trigger

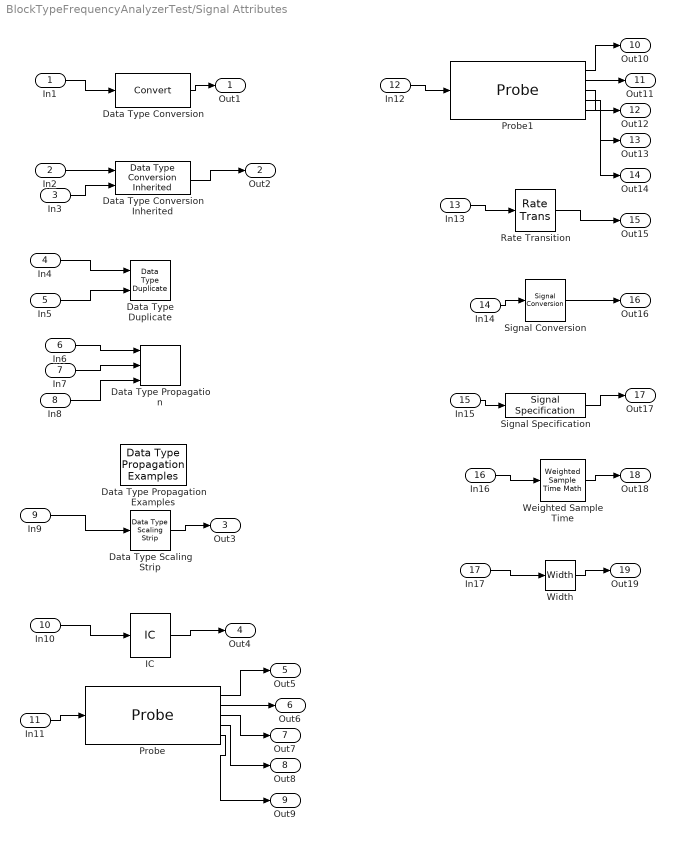
== system BlockTypeFrequencyAnalyzerTest/Signal Attributes ==
  In1 : Inport
  In2 : Inport  Port=2
  In3 : Inport  Port=3
  In4 : Inport  Port=4
  In5 : Inport  Port=5
  In6 : Inport  Port=6
  In7 : Inport  Port=7
  In8 : Inport  Port=8
  In9 : Inport  Port=9
  In10 : Inport  Port=10
  In11 : Inport  Port=11
  In12 : Inport  Port=12
  In13 : Inport  Port=13
  In14 : Inport  Port=14
  In15 : Inport  Port=15
  In16 : Inport  Port=16
  In17 : Inport  Port=17
  Data Type Conversion Inherited : simulink/Signal Attributes/Data Type Conversion Inherited  ConvertRealWorld=Real World Value  DoSatur=off
  Data Type Duplicate : simulink/Signal Attributes/Data Type Duplicate  NumInputPorts=2
  Data Type Propagation : simulink/Signal Attributes/Data Type Propagation  PropDataType=sfix(16)  IfRefDouble=double  IfRefSingle=single  IsSigned=IsSigned1 or IsSigned2  NumBitsBase=max([NumBits1 NumBits2])  NumBitsMult=1  NumBitsAdd=0  NumBitsAllowFinal=1:128  PropScaling=2^-10  ValuesUsedBestPrec=[5 -7]  SlopeBase=min([Slope1 Slope2])  SlopeMult=1  SlopeAdd=0  BiasBase=Bias1  BiasMult=1  BiasAdd=0
  Data Type Propagation Examples : simulink/Signal Attributes/Data Type Propagation Examples
  Data Type Scaling Strip : simulink/Signal Attributes/Data Type Scaling Strip
  Data Type Conversion : DataTypeConversion
  IC : InitialCondition
  Probe : Probe  ProbeSignalDimensions=on  ProbeFramedSignal=on
  Probe1 : Probe  ProbeSignalDimensions=on  ProbeFramedSignal=on
  Rate Transition : RateTransition
  Signal Conversion : SignalConversion  ConversionOutput=Contiguous copy
  Signal Specification : SignalSpecification
  Weighted Sample Time : simulink/Math Operations/Weighted Sample Time Math  TsampMathOp=Ts Only  weightValue=1.0  TsampMathImp=Online Calculations  DoSatur=off
  Width : Width
  Out1 : Outport
  Out2 : Outport  Port=2
  Out3 : Outport  Port=3
  Out4 : Outport  Port=4
  Out5 : Outport  Port=5
  Out6 : Outport  Port=6
  Out7 : Outport  Port=7
  Out8 : Outport  Port=8
  Out9 : Outport  Port=9
  Out10 : Outport  Port=10
  Out11 : Outport  Port=11
  Out12 : Outport  Port=12
  Out13 : Outport  Port=13
  Out14 : Outport  Port=14
  Out15 : Outport  Port=15
  Out16 : Outport  Port=16
  Out17 : Outport  Port=17
  Out18 : Outport  Port=18
  Out19 : Outport  Port=19
  wires:
  In1/1 -> Data Type Conversion/1
  Data Type Conversion/1 -> Out1/1
  In2/1 -> Data Type Conversion Inherited/1
  In3/1 -> Data Type Conversion Inherited/2
  Data Type Conversion Inherited/1 -> Out2/1
  In4/1 -> Data Type Duplicate/1
  In5/1 -> Data Type Duplicate/2
  In6/1 -> Data Type Propagation/1
  In7/1 -> Data Type Propagation/2
  In8/1 -> Data Type Propagation/3
  In9/1 -> Data Type Scaling Strip/1
  Data Type Scaling Strip/1 -> Out3/1
  In10/1 -> IC/1
  IC/1 -> Out4/1
  In11/1 -> Probe/1
  Probe/1 -> Out5/1
  Probe/2 -> Out6/1
  Probe/3 -> Out7/1
  Probe/4 -> Out8/1
  Probe/5 -> Out9/1
  In12/1 -> Probe1/1
  Probe1/1 -> Out10/1
  Probe1/2 -> Out11/1
  Probe1/3 -> Out12/1
  Probe1/4 -> Out13/1
  Probe1/5 -> Out14/1
  In13/1 -> Rate Transition/1
  Rate Transition/1 -> Out15/1
  In14/1 -> Signal Conversion/1
  Signal Conversion/1 -> Out16/1
  In15/1 -> Signal Specification/1
  Signal Specification/1 -> Out17/1
  In16/1 -> Weighted Sample Time/1
  Weighted Sample Time/1 -> Out18/1
  In17/1 -> Width/1
  Width/1 -> Out19/1

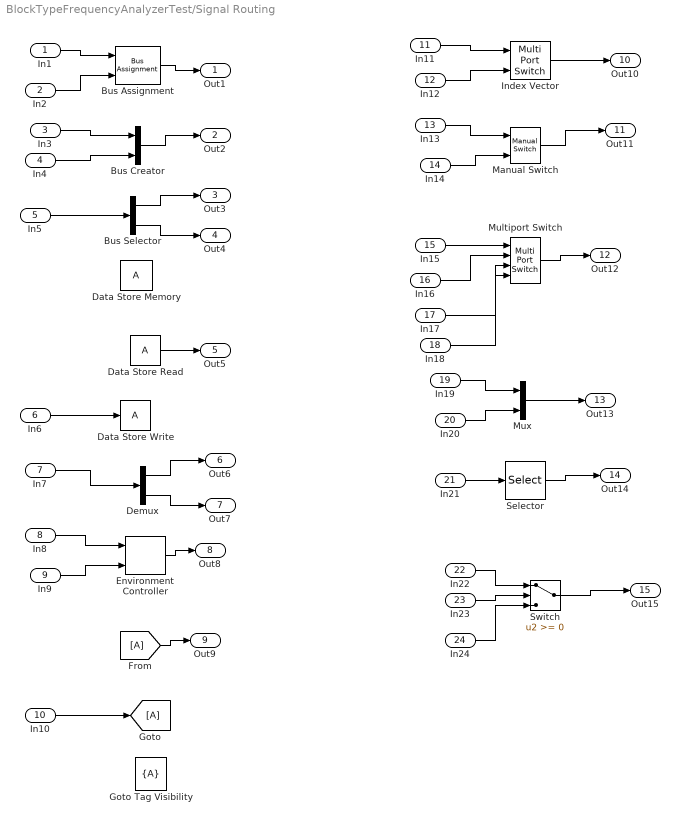
== system BlockTypeFrequencyAnalyzerTest/Signal Routing ==
  In1 : Inport
  In2 : Inport  Port=2
  In3 : Inport  Port=3
  In4 : Inport  Port=4
  In5 : Inport  Port=5
  In6 : Inport  Port=6
  In7 : Inport  Port=7
  In8 : Inport  Port=8
  In9 : Inport  Port=9
  In10 : Inport  Port=10
  In11 : Inport  Port=11
  In12 : Inport  Port=12
  In13 : Inport  Port=13
  In14 : Inport  Port=14
  In15 : Inport  Port=15
  In16 : Inport  Port=16
  In17 : Inport  Port=17
  In18 : Inport  Port=18
  In19 : Inport  Port=19
  In20 : Inport  Port=20
  In21 : Inport  Port=21
  In22 : Inport  Port=22
  In23 : Inport  Port=23
  In24 : Inport  Port=24
  Bus Assignment : BusAssignment
  Bus Creator : BusCreator  Inputs=2
  Bus Selector : BusSelector  OutputSignals=signal1,signal2
  Data Store Memory : DataStoreMemory  DataStoreName=A  ReadBeforeWriteMsg=warning  WriteAfterWriteMsg=warning  WriteAfterReadMsg=warning  InitialValue=0
  Data Store Read : DataStoreRead  DataStoreName=A  SampleTime=0
  Data Store Write : DataStoreWrite  DataStoreName=A  SampleTime=-1
  Demux : Demux  Outputs=2
  Environment Controller : simulink/Signal Routing/Environment Controller
  Goto Tag Visibility : GotoTagVisibility
  Index Vector : MultiPortSwitch  Inputs=1  zeroidx=on
  Manual Switch : simulink/Signal Routing/Manual Switch  sw=1  action=0
  Multiport Switch : MultiPortSwitch  Inputs=3
  Mux : Mux  Inputs=2
  Selector : Selector  Elements=[1 3]  InputPortWidth=3
  Switch : Switch
  Out1 : Outport
  Out2 : Outport  Port=2
  Out3 : Outport  Port=3
  Out4 : Outport  Port=4
  Out5 : Outport  Port=5
  Out6 : Outport  Port=6
  Out7 : Outport  Port=7
  Out8 : Outport  Port=8
  Out9 : Outport  Port=9
  Out10 : Outport  Port=10
  Out11 : Outport  Port=11
  Out12 : Outport  Port=12
  Out13 : Outport  Port=13
  Out14 : Outport  Port=14
  Out15 : Outport  Port=15
  wires:
  In1/1 -> Bus Assignment/1
  In2/1 -> Bus Assignment/2
  Bus Assignment/1 -> Out1/1
  In3/1 -> Bus Creator/1
  In4/1 -> Bus Creator/2
  Bus Creator/1 -> Out2/1
  In5/1 -> Bus Selector/1
  Bus Selector/1 -> Out3/1
  Bus Selector/2 -> Out4/1
  Data Store Read/1 -> Out5/1
  In6/1 -> Data Store Write/1
  In7/1 -> Demux/1
  Demux/1 -> Out6/1
  Demux/2 -> Out7/1
  In8/1 -> Environment Controller/1
  In9/1 -> Environment Controller/2
  Environment Controller/1 -> Out8/1
  [A] -> Out9/1
  In10/1 -> [A]
  In11/1 -> Index Vector/1
  In12/1 -> Index Vector/2
  Index Vector/1 -> Out10/1
  In13/1 -> Manual Switch/1
  In14/1 -> Manual Switch/2
  Manual Switch/1 -> Out11/1
  In15/1 -> Multiport Switch/1
  In16/1 -> Multiport Switch/2
  In17/1 -> Multiport Switch/3
  In18/1 -> Multiport Switch/4
  Multiport Switch/1 -> Out12/1
  In19/1 -> Mux/1
  In20/1 -> Mux/2
  Mux/1 -> Out13/1
  In21/1 -> Selector/1
  Selector/1 -> Out14/1
  In22/1 -> Switch/1
  In23/1 -> Switch/2
  In24/1 -> Switch/3
  Switch/1 -> Out15/1

== system BlockTypeFrequencyAnalyzerTest/Sinks ==
  In1 : Inport
  In2 : Inport  Port=2
  In3 : Inport  Port=3
  In4 : Inport  Port=4
  In5 : Inport  Port=5
  In6 : Inport  Port=6
  In7 : Inport  Port=7
  In8 : Inport  Port=8
  Display : Display
  Floating Scope : Scope
      settings: Floating=on
  Scope : Scope
      settings: SaveName=ScopeData2
  Stop Simulation : Stop
  Terminator : Terminator
  To File : ToFile
  To Workspace : ToWorkspace  VariableName=simout  SampleTime=-1  SaveFormat=Structure
  XY Graph : simulink/Sinks/XY Graph  xmin=-1  xmax=1  ymin=-1  ymax=1  st=-1
  wires:
  In1/1 -> Display/1
  In2/1 -> Scope/1
  In3/1 -> Stop Simulation/1
  In4/1 -> Terminator/1
  In5/1 -> To File/1
  In6/1 -> To Workspace/1
  In7/1 -> XY Graph/1
  In8/1 -> XY Graph/2

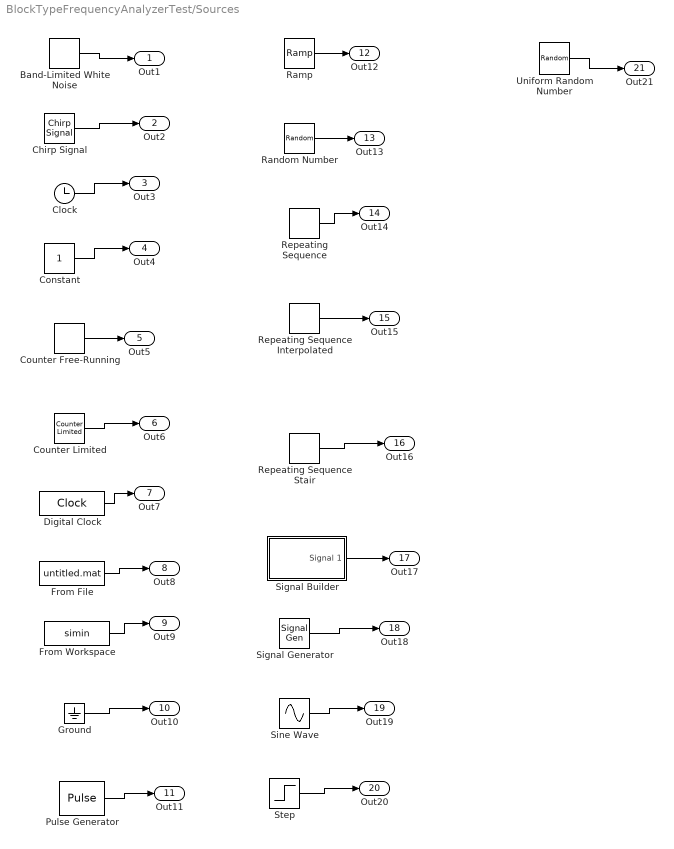
== system BlockTypeFrequencyAnalyzerTest/Sources ==
  Band-Limited White Noise : simulink/Sources/Band-Limited White Noise  Cov=[0.1]  Ts=0.1  seed=[23341]
  Chirp Signal : simulink/Sources/Chirp Signal  f1=0.1  T=100  f2=1
  Clock : Clock
      settings: Decimation=10
  Constant : Constant
  Counter Free-Running : simulink/Sources/Counter Free-Running  NumBits=16  tsamp=-1
  Counter Limited : simulink/Sources/Counter Limited  uplimit=7  tsamp=-1
  Digital Clock : DigitalClock
  From Workspace : FromWorkspace  VariableName=simin  SampleTime=0
  From File : FromFile  SampleTime=0
  Ground : Ground
  Pulse Generator : DiscretePulseGenerator  PulseType=Time based  PulseWidth=50
  Ramp : simulink/Sources/Ramp  slope=1  start=0  X0=0
  Random Number : RandomNumber  SampleTime=0
  Repeating Sequence : simulink/Sources/Repeating Sequence  rep_seq_t=[0 2]  rep_seq_y=[0 2]
  Repeating Sequence Interpolated : simulink/Sources/Repeating Sequence Interpolated  OutValues=[3 1 4 2 1].'  TimeValues=[0 0.1 0.5 0.6 1].'  LookUpMeth=Interpolation-Use End Values  tsamp=0.01  OutputDataTypeScalingMode=Specify via dialog  OutDataType=float('double')  OutScaling=2^-10
  Repeating Sequence Stair : simulink/Sources/Repeating Sequence Stair  OutValues=[3 1 4 2 1].'  tsamp=-1  OutputDataTypeScalingMode=Specify via dialog  OutDataType=float('double')  ConRadixGroup=Best Precision: Vector-wise  OutScaling=2^-12
  Signal Generator : SignalGenerator
  Signal Builder : Subsystem  Tag=STV Subsys  LoadFcn=sigbuilder_block('load');  StartFcn=sigbuilder_block('start');  StopFcn=sigbuilder_block('stop');  ClipboardFcn=sigbuilder_block('clipboard');  mask(Sigbuilder block){}
      mask help: Sigbuilder GUI
      mask init:
      | if ~strcmp(get_param(bdroot(gcbh),'SimulationStatus'),'stopped') tuvar = sigbuilder_block('maskInit'); end
      settings: CopyFcn=sigbuilder_block('copy');  DeleteFcn=sigbuilder_block('delete');  ModelCloseFcn=sigbuilder_block('modelClose');  PreSaveFcn=sigbuilder_block('preSave');  NameChangeFcn=sigbuilder_block('namechange');  OpenFcn=sigbuilder_block('open',[437.6 199.2 550.4 400 ]);  CloseFcn=sigbuilder_block('close');
      mask Display: plot(0,0,100,100,[10,10,40,40,10],[80,20,20,80,80],[40,10],[50,50], [40,27,10],[65,72,56],[40,25,25,10],[28,28,43,43]);
  Sine Wave : Sin  SampleTime=0
  Step : Step  SampleTime=0
  Uniform Random Number : UniformRandomNumber  SampleTime=0
  Out1 : Outport
  Out2 : Outport  Port=2
  Out3 : Outport  Port=3
  Out4 : Outport  Port=4
  Out5 : Outport  Port=5
  Out6 : Outport  Port=6
  Out7 : Outport  Port=7
  Out8 : Outport  Port=8
  Out9 : Outport  Port=9
  Out10 : Outport  Port=10
  Out11 : Outport  Port=11
  Out12 : Outport  Port=12
  Out13 : Outport  Port=13
  Out14 : Outport  Port=14
  Out15 : Outport  Port=15
  Out16 : Outport  Port=16
  Out17 : Outport  Port=17
  Out18 : Outport  Port=18
  Out19 : Outport  Port=19
  Out20 : Outport  Port=20
  Out21 : Outport  Port=21
  wires:
  Band-Limited White Noise/1 -> Out1/1
  Chirp Signal/1 -> Out2/1
  Clock/1 -> Out3/1
  Constant/1 -> Out4/1
  Counter Free-Running/1 -> Out5/1
  Counter Limited/1 -> Out6/1
  Digital Clock/1 -> Out7/1
  From File/1 -> Out8/1
  From Workspace/1 -> Out9/1
  Ground/1 -> Out10/1
  Pulse Generator/1 -> Out11/1
  Ramp/1 -> Out12/1
  Random Number/1 -> Out13/1
  Repeating Sequence/1 -> Out14/1
  Repeating Sequence Interpolated/1 -> Out15/1
  Repeating Sequence Stair/1 -> Out16/1
  Signal Builder/1(Signal 1) -> Out17/1
  Signal Generator/1 -> Out18/1
  Sine Wave/1 -> Out19/1
  Step/1 -> Out20/1
  Uniform Random Number/1 -> Out21/1

== system BlockTypeFrequencyAnalyzerTest/User-Defined Functions ==
  In1 : Inport
  In2 : Inport  Port=2
  In3 : Inport  Port=3
  In4 : Inport  Port=4
  In5 : Inport  Port=5
  In6 : Inport  Port=6
  Embedded MATLAB Function : Stateflow chart
  Fcn : Fcn  Expr=sin(u(1)*exp(2.3*(-u(2))))
  Level-2 M-file S-Function : M-S-Function
  MATLAB Fcn : MATLABFcn
  S-Function : S-Function
  S-Function Builder : S-Function  mask(S-Function Builder){}
      mask init:
      | val = [[.9  0.75 0.75 1 1 .9 .9 1]',[1 1 0.75 0.75 .9 .9 1 .9]'];
      | sys = get_param(gcbh,'FunctionName');
      settings: CopyFcn=set_param(gcbh,'LinkStatus','none')  OpenFcn=sfunctionwizard(gcbh)
      mask Display:
      | plot(val(:,1),val(:,2))
      | disp(sys)
  S-Function Examples : simulink/User-Defined Functions/S-Function Examples
  Out1 : Outport
  Out2 : Outport  Port=2
  Out3 : Outport  Port=3
  Out4 : Outport  Port=4
  Out5 : Outport  Port=5
  Out6 : Outport  Port=6
  wires:
  In1/1 -> Embedded MATLAB Function/1(u)
  Embedded MATLAB Function/1(y) -> Out1/1
  In2/1 -> Fcn/1
  Fcn/1 -> Out2/1
  In3/1 -> Level-2 M-file S-Function/1
  Level-2 M-file S-Function/1 -> Out3/1
  In4/1 -> MATLAB Fcn/1
  MATLAB Fcn/1 -> Out4/1
  In5/1 -> S-Function/1
  S-Function/1 -> Out5/1
  In6/1 -> S-Function Builder/1
  S-Function Builder/1 -> Out6/1

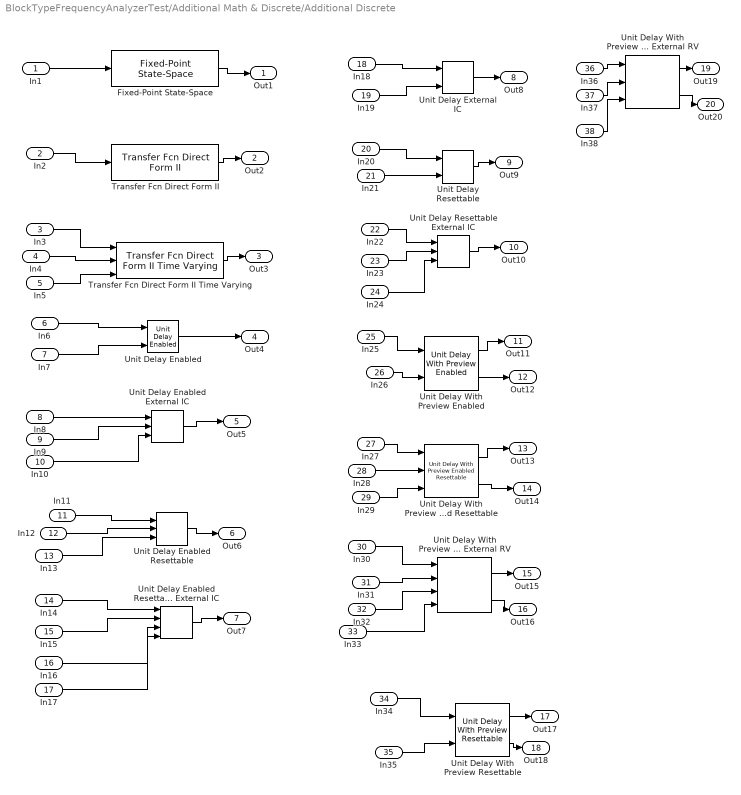
== system BlockTypeFrequencyAnalyzerTest/Additional Math & Discrete/Additional Discrete ==
  In1 : Inport
  In2 : Inport  Port=2
  In3 : Inport  Port=3
  In4 : Inport  Port=4
  In5 : Inport  Port=5
  In6 : Inport  Port=6
  In7 : Inport  Port=7
  In8 : Inport  Port=8
  In9 : Inport  Port=9
  In10 : Inport  Port=10
  In11 : Inport  Port=11
  In12 : Inport  Port=12
  In13 : Inport  Port=13
  In14 : Inport  Port=14
  In15 : Inport  Port=15
  In16 : Inport  Port=16
  In17 : Inport  Port=17
  In18 : Inport  Port=18
  In19 : Inport  Port=19
  In20 : Inport  Port=20
  In21 : Inport  Port=21
  In22 : Inport  Port=22
  In23 : Inport  Port=23
  In24 : Inport  Port=24
  In25 : Inport  Port=25
  In26 : Inport  Port=26
  In27 : Inport  Port=27
  In28 : Inport  Port=28
  In29 : Inport  Port=29
  In30 : Inport  Port=30
  In31 : Inport  Port=31
  In32 : Inport  Port=32
  In33 : Inport  Port=33
  In34 : Inport  Port=34
  In35 : Inport  Port=35
  In36 : Inport  Port=36
  In37 : Inport  Port=37
  In38 : Inport  Port=38
  Fixed-Point State-Space : simulink/Additional Math & Discrete/Additional Discrete/Fixed-Point State-Space  A=[2.6020 -2.2793 0.6708; 1 0 0; 0 1 0]  B=[ 1; 0; 0]  C="[0.0184    0.0024    0.0055]"  D=[0.0033]  X0=0.0  InternalDataType=float('double')  StateEqScaling=2^0  OutputEqScaling=2^0  DoSatur=off
  Transfer Fcn Direct Form II : simulink/Additional Math & Discrete/Additional Discrete/Transfer Fcn Direct Form II  NumCoefVec=[0.2 0.3 0.2]  DenCoefVec="[-0.9    0.6]"  vinit=0.0  DoSatur=off
  Transfer Fcn Direct Form II Time Varying : simulink/Additional Math & Discrete/Additional Discrete/Transfer Fcn Direct Form II Time Varying  vinit=0.0  DoSatur=off
  Unit Delay Enabled : simulink/Additional Math & Discrete/Additional Discrete/Unit Delay Enabled  vinit=0.0  tsamp=-1
  Unit Delay Enabled External IC : simulink/Additional Math & Discrete/Additional Discrete/Unit Delay Enabled External IC  tsamp=-1
  Unit Delay Enabled Resettable : simulink/Additional Math & Discrete/Additional Discrete/Unit Delay Enabled Resettable  vinit=0.0  tsamp=-1
  Unit Delay Enabled Resettable External IC : simulink/Additional Math & Discrete/Additional Discrete/Unit Delay Enabled Resettable External IC  tsamp=-1
  Unit Delay External IC : simulink/Additional Math & Discrete/Additional Discrete/Unit Delay External IC  tsamp=-1
  Unit Delay Resettable : simulink/Additional Math & Discrete/Additional Discrete/Unit Delay Resettable  vinit=0.0  tsamp=-1
  Unit Delay Resettable External IC : simulink/Additional Math & Discrete/Additional Discrete/Unit Delay Resettable External IC  tsamp=-1
  Unit Delay With Preview Enabled : simulink/Additional Math & Discrete/Additional Discrete/Unit Delay With Preview Enabled  vinit=0.0  tsamp=-1
  Unit Delay With Preview Enabled Resettable : simulink/Additional Math & Discrete/Additional Discrete/Unit Delay With Preview Enabled Resettable  vinit=0.0  tsamp=-1
  Unit Delay With Preview Enabled Resettable External RV : simulink/Additional Math & Discrete/Additional Discrete/Unit Delay With Preview Enabled Resettable External RV  vinit=0.0  tsamp=-1
  Unit Delay With Preview Resettable : simulink/Additional Math & Discrete/Additional Discrete/Unit Delay With Preview Resettable  vinit=0.0  tsamp=-1
  Unit Delay With Preview Resettable External RV : simulink/Additional Math & Discrete/Additional Discrete/Unit Delay With Preview Resettable External RV  vinit=0.0  tsamp=-1
  Out1 : Outport
  Out2 : Outport  Port=2
  Out3 : Outport  Port=3
  Out4 : Outport  Port=4
  Out5 : Outport  Port=5
  Out6 : Outport  Port=6
  Out7 : Outport  Port=7
  Out8 : Outport  Port=8
  Out9 : Outport  Port=9
  Out10 : Outport  Port=10
  Out11 : Outport  Port=11
  Out12 : Outport  Port=12
  Out13 : Outport  Port=13
  Out14 : Outport  Port=14
  Out15 : Outport  Port=15
  Out16 : Outport  Port=16
  Out17 : Outport  Port=17
  Out18 : Outport  Port=18
  Out19 : Outport  Port=19
  Out20 : Outport  Port=20
  wires:
  In1/1 -> Fixed-Point State-Space/1
  Fixed-Point State-Space/1 -> Out1/1
  In2/1 -> Transfer Fcn Direct Form II/1
  Transfer Fcn Direct Form II/1 -> Out2/1
  In3/1 -> Transfer Fcn Direct Form II Time Varying/1
  In4/1 -> Transfer Fcn Direct Form II Time Varying/2
  In5/1 -> Transfer Fcn Direct Form II Time Varying/3
  Transfer Fcn Direct Form II Time Varying/1 -> Out3/1
  In6/1 -> Unit Delay Enabled/1
  In7/1 -> Unit Delay Enabled/2
  Unit Delay Enabled/1 -> Out4/1
  In8/1 -> Unit Delay Enabled External IC/1
  In9/1 -> Unit Delay Enabled External IC/2
  In10/1 -> Unit Delay Enabled External IC/3
  Unit Delay Enabled External IC/1 -> Out5/1
  In11/1 -> Unit Delay Enabled Resettable/1
  In12/1 -> Unit Delay Enabled Resettable/2
  In13/1 -> Unit Delay Enabled Resettable/3
  Unit Delay Enabled Resettable/1 -> Out6/1
  In14/1 -> Unit Delay Enabled Resettable External IC/1
  In15/1 -> Unit Delay Enabled Resettable External IC/2
  In16/1 -> Unit Delay Enabled Resettable External IC/3
  In17/1 -> Unit Delay Enabled Resettable External IC/4
  Unit Delay Enabled Resettable External IC/1 -> Out7/1
  In18/1 -> Unit Delay External IC/1
  In19/1 -> Unit Delay External IC/2
  Unit Delay External IC/1 -> Out8/1
  In36/1 -> Unit Delay With Preview Resettable External RV/1
  In37/1 -> Unit Delay With Preview Resettable External RV/2
  In38/1 -> Unit Delay With Preview Resettable External RV/3
  Unit Delay With Preview Resettable External RV/1 -> Out19/1
  Unit Delay With Preview Resettable External RV/2 -> Out20/1
  In20/1 -> Unit Delay Resettable/1
  In21/1 -> Unit Delay Resettable/2
  Unit Delay Resettable/1 -> Out9/1
  In22/1 -> Unit Delay Resettable External IC/1
  In23/1 -> Unit Delay Resettable External IC/2
  In24/1 -> Unit Delay Resettable External IC/3
  Unit Delay Resettable External IC/1 -> Out10/1
  In25/1 -> Unit Delay With Preview Enabled/1
  In26/1 -> Unit Delay With Preview Enabled/2
  Unit Delay With Preview Enabled/1 -> Out11/1
  Unit Delay With Preview Enabled/2 -> Out12/1
  In27/1 -> Unit Delay With Preview Enabled Resettable/1
  In28/1 -> Unit Delay With Preview Enabled Resettable/2
  In29/1 -> Unit Delay With Preview Enabled Resettable/3
  Unit Delay With Preview Enabled Resettable/1 -> Out13/1
  Unit Delay With Preview Enabled Resettable/2 -> Out14/1
  In30/1 -> Unit Delay With Preview Enabled Resettable External RV/1
  In31/1 -> Unit Delay With Preview Enabled Resettable External RV/2
  In32/1 -> Unit Delay With Preview Enabled Resettable External RV/3
  In33/1 -> Unit Delay With Preview Enabled Resettable External RV/4
  Unit Delay With Preview Enabled Resettable External RV/1 -> Out15/1
  Unit Delay With Preview Enabled Resettable External RV/2 -> Out16/1
  In34/1 -> Unit Delay With Preview Resettable/1
  In35/1 -> Unit Delay With Preview Resettable/2
  Unit Delay With Preview Resettable/1 -> Out17/1
  Unit Delay With Preview Resettable/2 -> Out18/1

== system BlockTypeFrequencyAnalyzerTest/Additional Math & Discrete/Additional Math ==
  In1 : Inport
  In2 : Inport  Port=2
  In3 : Inport  Port=3
  In4 : Inport  Port=4
  In5 : Inport  Port=5
  In6 : Inport  Port=6
  Decrement Real World : simulink/Additional Math & Discrete/Additional Math: Increment - Decrement/Decrement Real World
  Decrement Stored Integer : simulink/Additional Math & Discrete/Additional Math: Increment - Decrement/Decrement Stored Integer
  Decrement To Zero : simulink/Additional Math & Discrete/Additional Math: Increment - Decrement/Decrement To Zero
  Decrement Time To Zero : simulink/Additional Math & Discrete/Additional Math: Increment - Decrement/Decrement Time To Zero
  Increment Real World : simulink/Additional Math & Discrete/Additional Math: Increment - Decrement/Increment Real World
  Increment Stored Integer : simulink/Additional Math & Discrete/Additional Math: Increment - Decrement/Increment Stored Integer
  Out2 : Outport
  Out3 : Outport  Port=2
  Out4 : Outport  Port=3
  Out5 : Outport  Port=4
  Out6 : Outport  Port=5
  Out7 : Outport  Port=6
  wires:
  In1/1 -> Decrement Real World/1
  Decrement Real World/1 -> Out2/1
  In2/1 -> Decrement Stored Integer/1
  Decrement Stored Integer/1 -> Out3/1
  In3/1 -> Decrement Time To Zero/1
  Decrement Time To Zero/1 -> Out4/1
  In4/1 -> Decrement To Zero/1
  Decrement To Zero/1 -> Out5/1
  In5/1 -> Increment Real World/1
  Increment Real World/1 -> Out6/1
  In6/1 -> Increment Stored Integer/1
  Increment Stored Integer/1 -> Out7/1

== system BlockTypeFrequencyAnalyzerTest/Commonly Used/Subsystem ==
  In1 : Inport
  Out1 : Outport
  wires:
  In1/1 -> Out1/1

== system BlockTypeFrequencyAnalyzerTest/Sources/Signal Builder ==
  Demux : Demux  Tag=STV Demux  Outputs=1
  FromWs : FromWorkspace  Tag=STV FromWs  VariableName=tuvar  SampleTime=0  SigBuilderData=DataTag0  VnvData=DataTag1
      SigBuilderData=|
      | channels.label = 'Signal 1'
      | channels.allXData = {[0 4 4 6 6 10]}
      | channels.allYData = {[0 0 1 1 0 0]}
      | common.afterFinalStr = 'Extrapolate'
      | common.sampleTime = 0
      | dataSet.timeRange = [0 10]
      | dataSet.name = 'Group 1'
  Signal 1 : Outport  Tag=STV Outport
  wires:
  Demux/1 -> Signal 1/1
  FromWs/1 -> Demux/1

== matlab function User-Defined Functions/Embedded MATLAB Function ==
  data: u input inherited; y output inherited
function y = fcn(u)
% This block supports an embeddable subset of the MATLAB language.
% See the help menu for details. 

y = u;
